simulink model "Copy_of_linkleg_trajectory_contact"  (R2022b)
settings: Solver=daessc  StartTime=0.0  StopTime=4  FixedStep=0.001  MaxStep=0.0025  RelTol=3e-3  AbsTol=3e-3  EnableMultiTasking=on
StopFcn:
  | Initialize = 0;
model workspace (MAT data in the model file):
  Initialize = Simulink.Signal
  Initialize.DataType = 'auto'
  Initialize.Dimensions = -1
  Initialize.DimensionsMode = 'auto'
  Initialize.Complexity = 'auto'
  Initialize.SampleTime = -1
  Initialize.SamplingMode = 'auto'
  Initialize.InitialValue = '0'
  Var = [0; 0; 0]
undefined symbols (not defined in the file or in its folder): X, Y, Z
libraries: sm_lib x86, nesl_utility x18, fl_lib x8, simulink x7, slpidlib x2, Contact_Forces_Lib x1
(part 1 of 3)
settings Model: SimulationMode=accelerator  Creator=guanlunlu  LastModifiedBy=guanlunlu
settings SolverCC: AutoScaleAbsTol=off  InitialStep=0.0025  MaxZcPerStep=1
settings DataIOCC: LimitDataPoints=on  MaxDataPoints=10000  LoggingToFile=on
settings OptimizationCC: DefaultParameterBehavior=Inlined  UseDivisionForNetSlopeComputation=on  GainParamInheritBuiltInType=on  UseFloatMulNetSlope=on  InlineInvariantSignals=on  EfficientFloat2IntCast=on  LifeSpan=1
settings DebuggingCC: UnconnectedInputMsg=warning  UnconnectedOutputMsg=warning  UnconnectedLineMsg=warning  AllowSymbolicDim=off  SFUnexpectedBacktrackingDiag=warning  SFNoUnconditionalDefaultTransitionDiag=warning  SFExecutionAtInitializationDiag=none  SFMachineParentedDataDiag=warning  ArithmeticOperatorsInVariantConditions=warning
settings HardwareCC: ProdLongLongMode=on
settings ModelReferenceCC: EnableRefExpFcnMdlSchedulingChecks=on
settings SFSimCC: SimUseLocalCustomCode=off  MATLABDynamicMemAlloc=off  CustomCodeUndefinedFunction=UseInterfaceOnly
settings RTWCC: GenerateReport=on  RTWUseLocalCustomCode=off  LaunchReport=on  DLArmComputeVersion=19.05
settings CodeAppCC: ForceParamTrailComments=on
settings GRTTargetCC: TargetLangStandard=C89/C90 (ANSI)  CombineSignalStateStructs=on  MatFileLogging=off  SupportVariableSizeSignals=on
settings ConfigComp: CovMetricSettings=dw  CovSaveCumulativeToWorkspaceVar=on  CovSaveSingleToWorkspaceVar=on  CovExternalEMLEnable=off  CovSFcnEnable=off
settings SimscapeCC: SimscapeLogType=all  SimscapeLogSimulationStatistics=on  SimscapeLogDataHistory=10000
settings ExplorerConfigSet: InternalSimMechanicsExplorerSettings="<ExplorerConfiguration><canonicalview>default</canonicalview><AnimationSetting><BasePlaybackSpeed>1.0</BasePlaybackSpeed><PlaybackSpeedFactor>1.0</PlaybackSpeedFactor></AnimationSetting><TilePanel><TileInfo><Tiles Columns=\"1\" Count=\"1\" Rows=\"1\"><Column Weight=\"1\"/><Row Weight=\"1\"/><Tile Height=\"1\" Width=\"1\" X=\"0\" Y=\"0\"/></Tiles></TileInfo><SceneInfo><SceneViewer><BGColor><R>1</R><G>1</G><B>1</B></BGColor><Camera><DoPerspective>off</DoPerspective><Position><X>0.000681433050903873516</X><Y>-0.0104115297967437362</Y><Z>1428355.60663242452</Z></Position><Center><X>0.000681433050903873516</X><Y>-0.0104115297967437362</Y><Z>2.07935910268020052e-07</Z></Center><Up><X>0</X><Y>1</Y><Z>-0</Z></Up><ViewLimDist>1</ViewLimDist><YLim>0.224878371170773472</YLim><XLim>0.312101415871202159</XLim></Camera></SceneViewer></SceneInfo></TilePanel><MechEditorPanel><Cameras/><GfxPanelCameraMap/><VideoCreator><PlaybackSpeedRatio>1.0</PlaybackSpeedRatio><FrameRate>30</FrameRate><VideoFormat>Motion JPEG AVI</VideoFormat><FrameSize>auto</FrameSize></VideoCreator></MechEditorPanel></ExplorerConfiguration>"

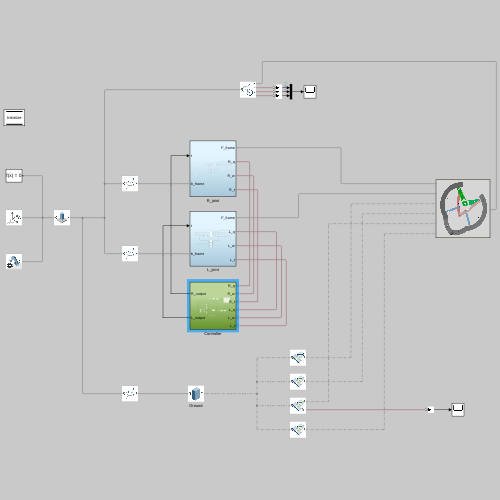
[thumbnail: Simulink's stored preview of the top-level diagram]
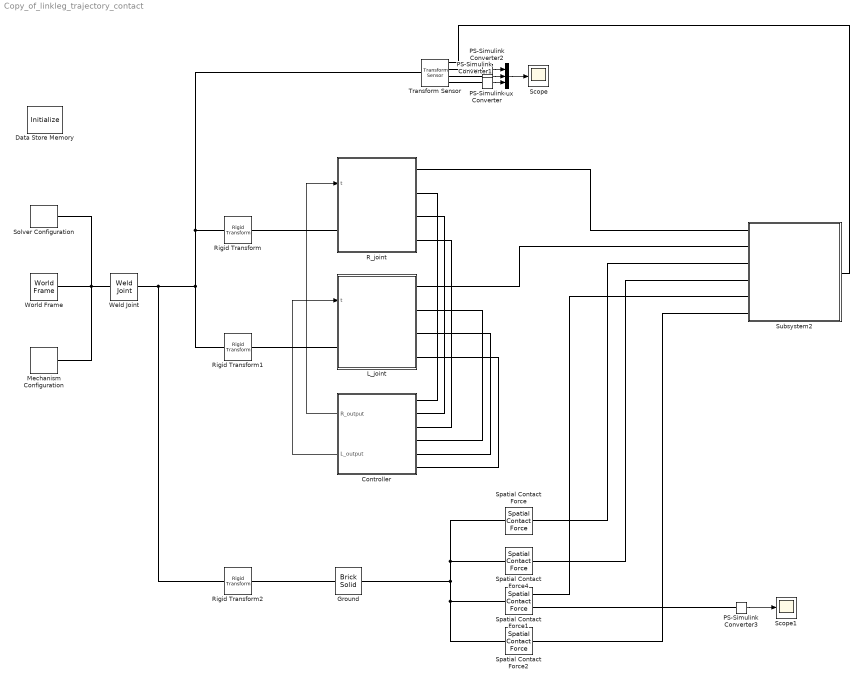
== system Copy_of_linkleg_trajectory_contact ==
  Controller : Subsystem
  Data Store Memory : DataStoreMemory  DataStoreName=Initialize  WriteAfterWriteMsg=warning  ShowAdditionalParam=off  StateMustResolveToSignalObject=on
  Ground : sm_lib/Body Elements/Brick Solid  GraphicAmbientColor=[0.15 0.15 0.15 1.0]  BasedOnType=Density  BrickDimensions=[1 1 0.02]  BrickDimensionUnits=m  CenterOfMass=[0 0 0]  CenterOfMassUnits=m  GraphicDiffuseColor=[1.0 0.8 0.8]  Density=1000  DensityUnits=kg/m^3  DoExposeReferenceFrame=on  GraphicEmissiveColor=[0.0 0.0 0.0 1.0]  ExportEntireGeometry=on  SerializedFrames=<Frames/>  MarkerShape=Sphere  MarkerSize=10  GraphicType=FromGeometry  InertiaType=CalculateFromGeometry  Mass=1  MassUnits=kg  MomentsOfInertia=[1 1 1]  MomentsOfInertiaUnits=kg*m^2  GraphicOpacity=1.0  ProductsOfInertia=[0 0 0]  ProductsOfInertiaUnits=kg*m^2  GraphicShininess=75  GraphicSpecularColor=[0.5 0.5 0.5 1.0]  GraphicVisPropType=SimpleVisualProperties
  L_joint : Subsystem
  Mechanism Configuration : sm_lib/Utilities/Mechanism Configuration  UniformGravity=Constant  GravityVector=[0 -9.80665 0]  GravityUnits=m/s^2  LinearizationDelta=0.001  JointModeTransitionNonlinearIterations=2
  Mux : Mux  Inputs=3
  PS-Simulink Converter{,1..3} (4 alike) : nesl_utility/PS-Simulink Converter  PhysicalDomain=network_engine_domain  SubClassName=ps_output  LeftPortType=input  RightPortType=output  PseudoPeriodic=off  Frequencies=[]  VectorFormat=inherit  Unit=inherit  AffineConversion=off
  R_joint : Subsystem
  Rigid Transform : sm_lib/Frames and Transforms/Rigid Transform  TranslationMethod=Cartesian  TranslationStandardOffset=0  TranslationLengthUnit=m  TranslationStandardAxis=+Z  TranslationCartesianOffset=[0 0 -0.005]  TranslationROffset=0  TranslationROffsetUnits=m  TranslationZOffset=0  TranslationZOffsetUnits=m  TranslationThetaOffset=0  TranslationThetaOffsetUnits=deg  RotationMethod=RotationSequence  RotationAngleUnits=deg  RotationStandardAxis=-Z  RotationAngle=0.0  RotationArbitraryAxis=[0 0 1]  FollAlignAxisA=+X  BaseAlignAxisA=+Y  FollAlignAxisB=+Y  BaseAlignAxisB=+Z  RotationSequenceAxes=FollowerAxes  RotationSequence=XYX  RotationSequenceAngles=[0 0 0]  RotationSequenceAnglesUnits=deg  RotationMatrix=[1 0 0; 0 1 0; 0 0 -1]  Quaternion=[1 0 0 0]
  Rigid Transform1 : sm_lib/Frames and Transforms/Rigid Transform  TranslationMethod=Cartesian  TranslationStandardOffset=0  TranslationLengthUnit=m  TranslationStandardAxis=+Z  TranslationCartesianOffset=[0 0 0.005]  TranslationROffset=0  TranslationROffsetUnits=m  TranslationZOffset=0  TranslationZOffsetUnits=m  TranslationThetaOffset=0  TranslationThetaOffsetUnits=deg  RotationMethod=None  RotationAngleUnits=deg  RotationStandardAxis=+Z  RotationAngle=0.0  RotationArbitraryAxis=[0 0 1]  FollAlignAxisA=+X  BaseAlignAxisA=+Y  FollAlignAxisB=+Y  BaseAlignAxisB=+Z  RotationSequenceAxes=FollowerAxes  RotationSequence=XYX  RotationSequenceAngles=[0 0 0]  RotationSequenceAnglesUnits=deg  RotationMatrix=[1 0 0; 0 1 0; 0 0 1]  Quaternion=[1 0 0 0]
  Rigid Transform2 : sm_lib/Frames and Transforms/Rigid Transform  TranslationMethod=Cartesian  TranslationStandardOffset=0  TranslationLengthUnit=m  TranslationStandardAxis=+Z  TranslationCartesianOffset=[0 -0.21 0]  TranslationROffset=0  TranslationROffsetUnits=m  TranslationZOffset=0  TranslationZOffsetUnits=m  TranslationThetaOffset=0  TranslationThetaOffsetUnits=deg  RotationMethod=StandardAxis  RotationAngleUnits=deg  RotationStandardAxis=-X  RotationAngle=90  RotationArbitraryAxis=[0 0 1]  FollAlignAxisA=+X  BaseAlignAxisA=+Y  FollAlignAxisB=+Y  BaseAlignAxisB=+Z  RotationSequenceAxes=FollowerAxes  RotationSequence=XYX  RotationSequenceAngles=[0 0 0]  RotationSequenceAnglesUnits=deg  RotationMatrix=[1 0 0; 0 1 0; 0 0 1]  Quaternion=[1 0 0 0]
  Scope : Scope
  Scope1 : Scope
  Solver Configuration : nesl_utility/Solver Configuration  PhysicalDomain=network_engine_domain  SubClassName=solver  LeftPortType=input  RightPortType=generic  Tones=[]  Harmonics=[]  SimulateNoise=off  Profile=off  UseLocalSampling=off  EnableSwitchedLinearOptims=on  FrequencyDomain=off  UseCCode=off  RelTol=0.001  AbsTol=1e-06  MinStep=1e-09  ToWorkspace=off  RevertToSquareIcSolve=off  NumHomotopyIterations=100  PhasorMode=off  PhasorModeNumHarmonics=1  ConsistencySolver=NEWTON_XTOL_AFTER_FTOL  IndexReductionMethod=DerivativeReplacement  DoDC=off  ResidualTolerance=1e-09  ConsistencyTolSource=GLOBAL  ConsistencyAbsTol=0.001  ConsistencyRelTol=0.001  ConsistencyTolFactor=0.001  UseLocalSolver=off  LocalSolverChoice=NE_BACKWARD_EULER_ADVANCER  ResolveIndetEquations=on  FunctionEvalNumThread=1  LocalSolverSampleTime=0.001  DoFixedCost=off  MaxNonlinIter=3  MaxModeIter=2  ComputeImpulses=off  ImpulseIterations=2  LinearAlgebra=Sparse  LinearAlgebraNumThread=0  EquationFormulation=NE_TIME_EF  DelaysMemoryBudget=1024  AutomaticFiltering=on  FilteringTimeConstant=0.001  PartitionStorageMethod=AS_NEEDED  PartitionMemoryBudget=1024  PartitionMethod=FAST
  Spatial Contact Force : sm_lib/Forces and Torques/Spatial Contact Force  SenseContactBaseRotation=off  SenseContactBaseTranslation=off  CoefficientOfDynamicFriction=0.2  CoefficientOfStaticFriction=0.2  NormalDamping=contact_dmp  NormalDampingUnits=N/(m/s)  SenseContactSignal=off  NormalStiffness=contact_stf  NormalStiffnessUnits=N/m  FrictionalCriticalVelocity=1e-3  FrictionalCriticalVelocityUnits=m/s  ZeroCrossDetectContactStartAndEnd=off  SenseContactFollowerRotation=off  SenseContactFollowerTranslation=off  FrictionType=SmoothStickSlip  SenseFrictionalForceMagnitude=off  SenseNormalForceMagnitude=off  NormalForceType=SmoothSpringDamper  SenseNormalVelocity=off  SenseSeparationDistance=off  SenseTangentialVelocity=off  NormalTransitionRegionWidth=contact_trs  NormalTransitionRegionWidthUnits=m
  Spatial Contact Force1 : sm_lib/Forces and Torques/Spatial Contact Force  SenseContactBaseRotation=off  SenseContactBaseTranslation=off  CoefficientOfDynamicFriction=0.2  CoefficientOfStaticFriction=0.2  NormalDamping=contact_dmp  NormalDampingUnits=N/(m/s)  SenseContactSignal=off  NormalStiffness=contact_stf  NormalStiffnessUnits=N/m  FrictionalCriticalVelocity=1e-3  FrictionalCriticalVelocityUnits=m/s  ZeroCrossDetectContactStartAndEnd=off  SenseContactFollowerRotation=off  SenseContactFollowerTranslation=off  FrictionType=SmoothStickSlip  SenseFrictionalForceMagnitude=off  SenseNormalForceMagnitude=on  NormalForceType=SmoothSpringDamper  SenseNormalVelocity=off  SenseSeparationDistance=off  SenseTangentialVelocity=off  NormalTransitionRegionWidth=contact_trs  NormalTransitionRegionWidthUnits=m
  Spatial Contact Force2 : sm_lib/Forces and Torques/Spatial Contact Force  SenseContactBaseRotation=off  SenseContactBaseTranslation=off  CoefficientOfDynamicFriction=0.2  CoefficientOfStaticFriction=0.2  NormalDamping=contact_dmp  NormalDampingUnits=N/(m/s)  SenseContactSignal=off  NormalStiffness=contact_stf  NormalStiffnessUnits=N/m  FrictionalCriticalVelocity=1e-3  FrictionalCriticalVelocityUnits=m/s  ZeroCrossDetectContactStartAndEnd=off  SenseContactFollowerRotation=off  SenseContactFollowerTranslation=off  FrictionType=SmoothStickSlip  SenseFrictionalForceMagnitude=off  SenseNormalForceMagnitude=off  NormalForceType=SmoothSpringDamper  SenseNormalVelocity=off  SenseSeparationDistance=off  SenseTangentialVelocity=off  NormalTransitionRegionWidth=contact_trs  NormalTransitionRegionWidthUnits=m
  Spatial Contact Force4 : sm_lib/Forces and Torques/Spatial Contact Force  SenseContactBaseRotation=off  SenseContactBaseTranslation=off  CoefficientOfDynamicFriction=0.2  CoefficientOfStaticFriction=0.2  NormalDamping=contact_dmp  NormalDampingUnits=N/(m/s)  SenseContactSignal=off  NormalStiffness=contact_stf  NormalStiffnessUnits=N/m  FrictionalCriticalVelocity=1e-3  FrictionalCriticalVelocityUnits=m/s  ZeroCrossDetectContactStartAndEnd=off  SenseContactFollowerRotation=off  SenseContactFollowerTranslation=off  FrictionType=SmoothStickSlip  SenseFrictionalForceMagnitude=off  SenseNormalForceMagnitude=off  NormalForceType=SmoothSpringDamper  SenseNormalVelocity=off  SenseSeparationDistance=off  SenseTangentialVelocity=off  NormalTransitionRegionWidth=contact_trs  NormalTransitionRegionWidthUnits=m
  Subsystem2 : Subsystem
      mask Display: image('$imagefile'); % Use "Edit Image" on toolstrip to change.
  Transform Sensor : sm_lib/Frames and Transforms/Transform Sensor  MeasurementFrame=World  SenseAngle=off  SenseAxis=off  SenseQ=off  SenseR=off  SenseRotationSequence=off  RotationSequence=XYX  SenseOmegaX=off  SenseOmegaY=off  SenseOmegaZ=off  SenseQDot=off  SenseRDot=off  SenseAlphaX=off  SenseAlphaY=off  SenseAlphaZ=off  SenseQDDot=off  SenseRDDot=off  SenseX=on  SenseY=on  SenseZ=on  SenseRad=off  SenseAzim=off  SenseDist=off  SenseInc=off  SenseXDot=off  SenseYDot=off  SenseZDot=off  SenseRadDot=off  SenseAzimDot=off  SenseDistDot=off  SenseIncDot=off  SenseXDDot=off  SenseYDDot=off  SenseZDDot=off  SenseRadDDot=off  SenseAzimDDot=off  SenseDistDDot=off  SenseIncDDot=off
  Weld Joint : sm_lib/Joints/Weld Joint  JointMode=Normal  SenseConstraintForce=off  SenseConstraintForceX=off  SenseConstraintForceY=off  SenseConstraintForceZ=off  SenseConstraintTorque=off  SenseConstraintTorqueX=off  SenseConstraintTorqueY=off  SenseConstraintTorqueZ=off  SenseTotalForce=off  SenseTotalForceX=off  SenseTotalForceY=off  SenseTotalForceZ=off  SenseTotalTorque=off  SenseTotalTorqueX=off  SenseTotalTorqueY=off  SenseTotalTorqueZ=off  CompositeWrenchDir=FollowerOnBase  CompositeWrenchFrame=BaseFrame
  World Frame : sm_lib/Frames and Transforms/World Frame
  wires:
  Controller/1(R_output) -> R_joint/1(t)
  Controller/2(L_output) -> L_joint/1(t)
  Mux/1 -> Scope/1
  PS-Simulink Converter2/1 -> Mux/1
  PS-Simulink Converter1/1 -> Mux/3
  PS-Simulink Converter/1 -> Mux/2
  PS-Simulink Converter3/1 -> Scope1/1
  connections:
  World Frame/RConn1 -- Mechanism Configuration/RConn1 -- Weld Joint/LConn1 -- Solver Configuration/RConn1
  Rigid Transform/LConn1 -- Transform Sensor/LConn1 -- Rigid Transform1/LConn1 -- Rigid Transform2/LConn1 -- Weld Joint/RConn1
  Ground/RConn1 -- Rigid Transform2/RConn1
  R_joint/LConn1 -- Rigid Transform/RConn1
  Rigid Transform1/RConn1 -- L_joint/LConn1
  R_joint/RConn1 -- Subsystem2/LConn1
  L_joint/RConn1 -- Subsystem2/LConn2
  Spatial Contact Force/LConn1 -- Spatial Contact Force4/LConn1 -- Spatial Contact Force2/LConn1 -- Spatial Contact Force1/LConn1 -- Ground/LConn1
  Spatial Contact Force4/RConn1 -- Subsystem2/LConn4
  Spatial Contact Force/RConn1 -- Subsystem2/LConn3
  Spatial Contact Force1/RConn1 -- Subsystem2/LConn5
  Spatial Contact Force2/RConn1 -- Subsystem2/LConn6
  R_joint/RConn2 -- Controller/LConn1
  R_joint/RConn3 -- Controller/LConn2
  R_joint/RConn4 -- Controller/LConn3
  L_joint/RConn2 -- Controller/LConn4
  L_joint/RConn3 -- Controller/LConn5
  L_joint/RConn4 -- Controller/LConn6
  Transform Sensor/RConn1 -- Subsystem2/RConn1
  PS-Simulink Converter2/LConn1 -- Transform Sensor/RConn2
  Transform Sensor/RConn3 -- PS-Simulink Converter/LConn1
  Transform Sensor/RConn4 -- PS-Simulink Converter1/LConn1
  PS-Simulink Converter3/LConn1 -- Spatial Contact Force1/RConn2

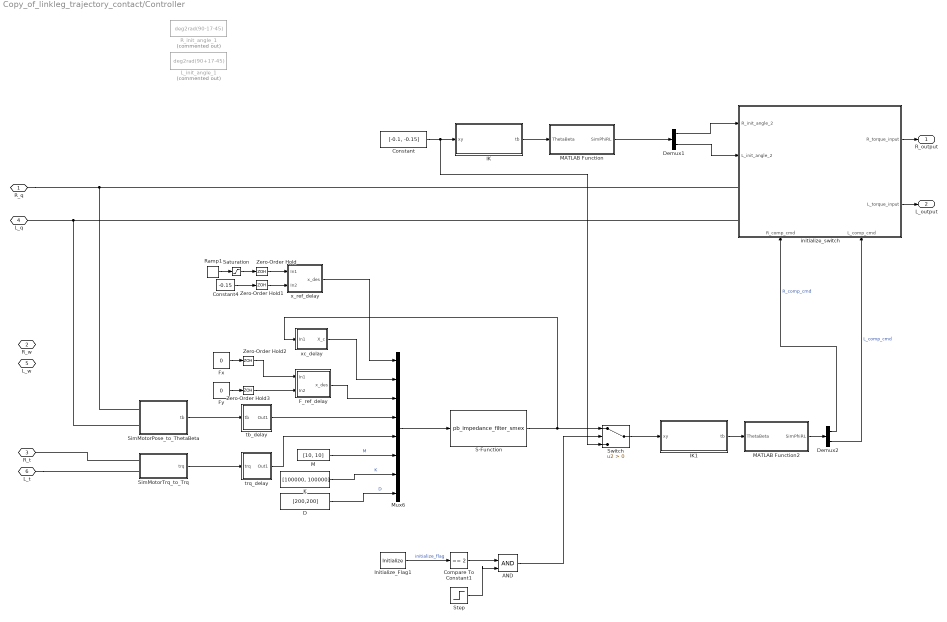
== system Copy_of_linkleg_trajectory_contact/Controller ==
  AND : Logic  IconShape=distinctive  AllPortsSameDT=off  OutDataTypeStr=boolean
  Compare To Constant1 : simulink/Logic and Bit Operations/Compare To Constant  relop===  const=2  OutDataTypeStr=uint8
  Constant : Constant  Value=[-0.1, -0.15]
  Constant4 : Constant  Value=-0.15
  D : Constant  Value=[200,200]
  Demux1 : Demux  Outputs=2
  Demux2 : Demux  Outputs=2
  F_ref_delay : Subsystem
  Fx : Constant  Value=0
  Fy : Constant  Value=0
  IK : MATLAB Function  TreatAsAtomicUnit=on
  IK1 : MATLAB Function  TreatAsAtomicUnit=on
  Initialize_Flag1 : DataStoreRead  DataStoreName=Initialize  IndexOptions=Index vector (dialog)  Indices=1  OutputSizes=1
  K : Constant  Value=[100000, 100000]
  L_init_angle_1 : Constant  Commented=on  Value=deg2rad(90+17-45)
  M : Constant  Value=[10, 10]
  MATLAB Function : MATLAB Function  TreatAsAtomicUnit=on
  MATLAB Function2 : MATLAB Function  TreatAsAtomicUnit=on
  Mux6 : Mux  Inputs=8
  R_init_angle_1 : Constant  Commented=on  Value=deg2rad(90-17-45)
  Ramp1 : simulink/Sources/Ramp  slope=0.1  start=1  InitialOutput=-0.1
  S-Function : S-Function  FunctionName=pb_impedance_filter_smex  SFunctionDeploymentMode=off  EnableBusSupport=off
  Saturation : Saturate  UpperLimit=0.1
  SimMotorPose_to_ThetaBeta : Subsystem
  SimMotorTrq_to_Trq : Subsystem
  Step : Step  SampleTime=0
  Switch : Switch  Criteria=u2 > Threshold  SaturateOnIntegerOverflow=off  InputSameDT=off
  Zero-Order Hold{,1..3} (4 alike) : ZeroOrderHold  SampleTime=-1
  initialize_switch : Subsystem
      settings: PortSchema="{\"entries\":[{\"content\":{\"sides\":[{\"content\":{\"connectorIds\":[\"In1\",\"In2\",\"LConn1\",\"LConn2\"]},\"type\":\"ConnectorPlacement.EquallySpacedRectSide\",\"uuid\":\"90e40c7c-5865-4836-be41-da90a1037084\"},{\"content\":{\"connectorIds\":[\"Out1\",\"Out2\"],\"side\":\"RIGHT\"},\"type\":\"ConnectorPlacement.EquallySpacedRectSide\",\"uuid\":\"b839b53b-6c19-45bc-b89b-7b093b626138\"},{\"content\":{\"connectorIds\":[],\"side\":\"TOP\"},\"type\":\"ConnectorPlacement.EquallySpacedRectSide\",\"uuid\":\"45e31397-8701-4b08-8e72-be675cbdf183\"},{\"content\":{\"connectorIds\":[\"In3\",\"In4\"],\"side\":\"BOTTOM\"},\"type\":\"ConnectorPlacement.EquallySpacedRectSide\",\"uuid\":\"48276d5b-6512-4d04-ace7-a3d739604563\"}]},\"type\":\"ConnectorPlacement.EquallySpacedConnector\",\"uuid\":\"ed524fdc-357c-4d9e-8bf8-882e26daba64\"}],\"packageUris\":[\"http://schema.mathworks.com/mf0/Connector/R2020b\"],\"version\":\"1.0\"}"
  tb_delay : Subsystem
  trq_delay : Subsystem
  x_ref_delay : Subsystem
  xc_delay : Subsystem
  R_q : PMIOPort  Side=Left
  R_w : PMIOPort  Port=2  Side=Left
  R_t : PMIOPort  Port=3  Side=Left
  L_q : PMIOPort  Port=4  Side=Left
  L_w : PMIOPort  Port=5  Side=Left
  L_t : PMIOPort  Port=6  Side=Left
  R_output : Outport
  L_output : Outport  Port=2
  wires:
  initialize_switch/2(L_torque_input) -> L_output/1
  Demux1/2 -> initialize_switch/2(L_init_angle_2)
  initialize_switch/1(R_torque_input) -> R_output/1
  Demux1/1 -> initialize_switch/1(R_init_angle_2)
  Constant/1 -> Switch/3, IK/1(xy)
  IK/1(tb) -> MATLAB Function/1(ThetaBeta)
  MATLAB Function/1(SimPhiRL) -> Demux1/1
  Fy/1 -> Zero-Order Hold3/1
  Ramp1/1 -> Saturation/1
  tb_delay/1(Out1) -> Mux6/4
  MATLAB Function2/1(SimPhiRL) -> Demux2/1
  Mux6/1 -> S-Function/1
  IK1/1(tb) -> MATLAB Function2/1(ThetaBeta)
  Fx/1 -> Zero-Order Hold2/1
  F_ref_delay/1(x_des) -> Mux6/3
  trq_delay/1(Out1) -> Mux6/5
  x_ref_delay/1(x_des) -> Mux6/1
  K/1 -> Mux6/7  "K"
  M/1 -> Mux6/6  "M"
  Constant4/1 -> Zero-Order Hold1/1
  D/1 -> Mux6/8  "D"
  xc_delay/1(X_c) -> Mux6/2
  Demux2/1 -> initialize_switch/3(R_comp_cmd)  "R_comp_cmd"
  Demux2/2 -> initialize_switch/4(L_comp_cmd)  "L_comp_cmd"
  SimMotorPose_to_ThetaBeta/1(tb) -> tb_delay/1(tb)
  SimMotorTrq_to_Trq/1(trq) -> trq_delay/1(trq)
  S-Function/1 -> xc_delay/1(In1), Switch/1
  AND/1 -> Switch/2
  Switch/1 -> IK1/1(xy)
  Step/1 -> AND/2
  Initialize_Flag1/1 -> Compare To Constant1/1  "initialize_flag"
  Compare To Constant1/1 -> AND/1
  Zero-Order Hold/1 -> x_ref_delay/1(In1)
  Zero-Order Hold1/1 -> x_ref_delay/2(In2)
  Zero-Order Hold2/1 -> F_ref_delay/1(In1)
  Zero-Order Hold3/1 -> F_ref_delay/2(In2)
  Saturation/1 -> Zero-Order Hold/1
  connections:
  R_q/RConn1 -- SimMotorPose_to_ThetaBeta/LConn1 -- initialize_switch/LConn1
  initialize_switch/LConn2 -- SimMotorPose_to_ThetaBeta/LConn2 -- L_q/RConn1
  L_t/RConn1 -- SimMotorTrq_to_Trq/LConn2
  SimMotorTrq_to_Trq/LConn1 -- R_t/RConn1

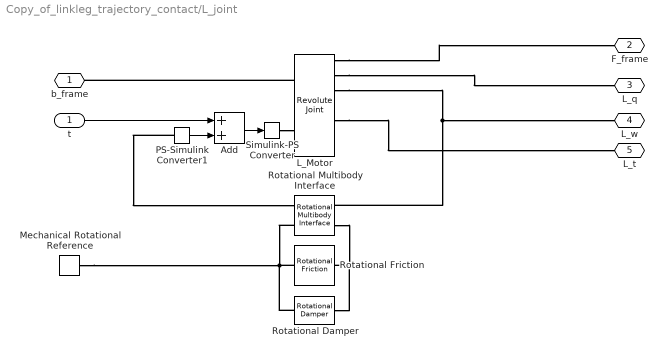
== system Copy_of_linkleg_trajectory_contact/L_joint ==
  t : Inport
  Add : Sum
  L_Motor : sm_lib/Joints/Revolute Joint  JointMode=Normal  SenseConstraintForce=on  SenseConstraintForceX=off  SenseConstraintForceY=off  SenseConstraintForceZ=off  SenseConstraintTorque=on  SenseConstraintTorqueX=off  SenseConstraintTorqueY=off  SenseConstraintTorqueZ=off  SenseTotalForce=off  SenseTotalForceX=off  SenseTotalForceY=off  SenseTotalForceZ=off  SenseTotalTorque=off  SenseTotalTorqueX=off  SenseTotalTorqueY=off  SenseTotalTorqueZ=off  CompositeWrenchDir=FollowerOnBase  CompositeWrenchFrame=BaseFrame  EquilibriumPosition=0  EquilibriumPositionUnits=deg  SpringStiffness=0  SpringStiffnessUnits=N*m/deg  DampingCoefficient=0  DampingCoefficientUnits=N*m/(rad/s)  TorqueActuationMode=InputTorque  MotionActuationMode=ComputedMotion  SensePosition=on  SenseVelocity=on  SenseAcceleration=on  SenseTorqueForce=on  SenseLowerLimitTorqueForce=off  SenseUpperLimitTorqueForce=off  LowerLimitSpecify=off  LowerLimitBound=-90  LowerLimitBoundUnits=deg  LowerLimitStiffness=1e4  LowerLimitStiffnessUnits=N*m/deg  LowerLimitDamping=10  LowerLimitDampingUnits=N*m/(deg/s)  LowerLimitTransitionRegionWidth=0.1  LowerLimitTransitionRegionWidthUnits=deg  UpperLimitSpecify=off  UpperLimitBound=90  UpperLimitBoundUnits=deg  UpperLimitStiffness=1e4  UpperLimitStiffnessUnits=N*m/deg  UpperLimitDamping=10  UpperLimitDampingUnits=N*m/(deg/s)  UpperLimitTransitionRegionWidth=0.1  UpperLimitTransitionRegionWidthUnits=deg  PositionTargetSpecify=on  PositionTargetPriority=High  PositionTargetValue=160  PositionTargetValueUnits=deg  VelocityTargetSpecify=off  VelocityTargetPriority=High  VelocityTargetValue=0  VelocityTargetValueUnits=deg/s
  Mechanical Rotational Reference : fl_lib/Mechanical/Rotational Elements/Mechanical Rotational Reference
  PS-Simulink Converter1 : nesl_utility/PS-Simulink Converter  PhysicalDomain=network_engine_domain  SubClassName=ps_output  LeftPortType=input  RightPortType=output  PseudoPeriodic=off  Frequencies=[]  VectorFormat=inherit  Unit=inherit  AffineConversion=off
  Rotational Damper : fl_lib/Mechanical/Rotational Elements/Rotational Damper  D=0.05 N*m*s/rad  w_specify=off  w_priority=None  w=0 rad/s  w_nominal_specify=off  w_nominal_unit=rad/s  w_nominal_value=1  t_specify=off  t_priority=None  t=0 N*m  t_nominal_specify=off  t_nominal_unit=N*m  t_nominal_value=1
  Rotational Friction : fl_lib/Mechanical/Rotational Elements/Rotational Friction  brkwy_trq=bk_ft N*m  brkwy_vel=bk_vel rad/s  Col_trq=col_ft N*m  visc_coef=vis_ft N*m*s/rad  w_specify=on  w_priority=None  w=0 rad/s  w_nominal_specify=off  w_nominal_unit=rad/s  w_nominal_value=1  t_specify=on  t_priority=None  t=0 N*m  t_nominal_specify=off  t_nominal_unit=N*m  t_nominal_value=1
  Rotational Multibody Interface : fl_lib/Mechanical/Multibody Interfaces/Rotational Multibody Interface
  Simulink-PS Converter : nesl_utility/Simulink-PS Converter  PhysicalDomain=network_engine_domain  SubClassName=ps_input  LeftPortType=input  RightPortType=output  PseudoPeriodic=off  Frequencies=[]  NoiseDistribution=none  NoiseParameters=[]  Unit=1  AffineConversion=off  FilteringAndDerivatives=provide  SimscapeFilterOrder=1  InputFilterTimeConstant=0.001  UdotUserProvided=0
  b_frame : PMIOPort  Side=Left
  F_frame : PMIOPort  Port=2  Side=Right
  L_q : PMIOPort  Port=3  Side=Right
  L_w : PMIOPort  Port=4  Side=Right
  L_t : PMIOPort  Port=5  Side=Right
  wires:
  PS-Simulink Converter1/1 -> Add/2
  Add/1 -> Simulink-PS Converter/1
  t/1 -> Add/1
  connections:
  PS-Simulink Converter1/LConn1 -- Rotational Multibody Interface/LConn1
  L_Motor/RConn1 -- F_frame/RConn1
  L_Motor/LConn1 -- b_frame/RConn1
  Rotational Multibody Interface/RConn2 -- Rotational Damper/LConn1 -- Rotational Friction/LConn1
  Simulink-PS Converter/RConn1 -- L_Motor/LConn2
  Rotational Multibody Interface/LConn2 -- Mechanical Rotational Reference/LConn1 -- Rotational Damper/RConn1 -- Rotational Friction/RConn1
  L_Motor/RConn3 -- L_w/RConn1 -- Rotational Multibody Interface/RConn1
  L_Motor/RConn2 -- L_q/RConn1
  L_Motor/RConn5 -- L_t/RConn1

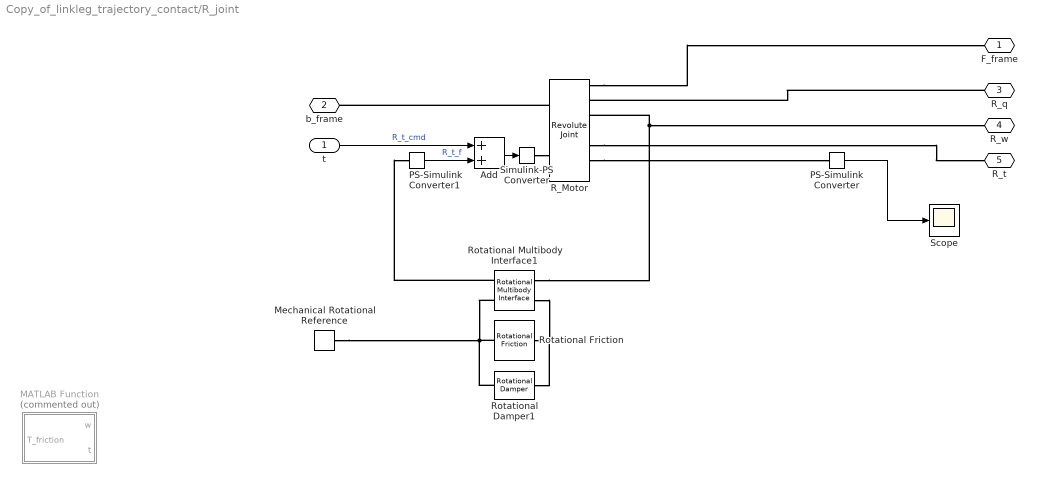
== system Copy_of_linkleg_trajectory_contact/R_joint ==
  t : Inport
  Add : Sum
  MATLAB Function : MATLAB Function  Commented=on  TreatAsAtomicUnit=on
  Mechanical Rotational Reference : fl_lib/Mechanical/Rotational Elements/Mechanical Rotational Reference
  PS-Simulink Converter : nesl_utility/PS-Simulink Converter  PhysicalDomain=network_engine_domain  SubClassName=ps_output  LeftPortType=input  RightPortType=output  PseudoPeriodic=off  Frequencies=[]  VectorFormat=inherit  Unit=inherit  AffineConversion=off
  PS-Simulink Converter1 : nesl_utility/PS-Simulink Converter  PhysicalDomain=network_engine_domain  SubClassName=ps_output  LeftPortType=input  RightPortType=output  PseudoPeriodic=off  Frequencies=[]  VectorFormat=inherit  Unit=inherit  AffineConversion=off
  R_Motor : sm_lib/Joints/Revolute Joint  JointMode=Normal  SenseConstraintForce=on  SenseConstraintForceX=off  SenseConstraintForceY=off  SenseConstraintForceZ=off  SenseConstraintTorque=on  SenseConstraintTorqueX=off  SenseConstraintTorqueY=off  SenseConstraintTorqueZ=off  SenseTotalForce=off  SenseTotalForceX=off  SenseTotalForceY=off  SenseTotalForceZ=off  SenseTotalTorque=off  SenseTotalTorqueX=off  SenseTotalTorqueY=off  SenseTotalTorqueZ=off  CompositeWrenchDir=FollowerOnBase  CompositeWrenchFrame=BaseFrame  EquilibriumPosition=0  EquilibriumPositionUnits=deg  SpringStiffness=0  SpringStiffnessUnits=N*m/deg  DampingCoefficient=0  DampingCoefficientUnits=N*m/(rad/s)  TorqueActuationMode=InputTorque  MotionActuationMode=ComputedMotion  SensePosition=on  SenseVelocity=on  SenseAcceleration=on  SenseTorqueForce=on  SenseLowerLimitTorqueForce=off  SenseUpperLimitTorqueForce=off  LowerLimitSpecify=off  LowerLimitBound=-90  LowerLimitBoundUnits=deg  LowerLimitStiffness=1e4  LowerLimitStiffnessUnits=N*m/deg  LowerLimitDamping=10  LowerLimitDampingUnits=N*m/(deg/s)  LowerLimitTransitionRegionWidth=0.1  LowerLimitTransitionRegionWidthUnits=deg  UpperLimitSpecify=off  UpperLimitBound=90  UpperLimitBoundUnits=deg  UpperLimitStiffness=1e4  UpperLimitStiffnessUnits=N*m/deg  UpperLimitDamping=10  UpperLimitDampingUnits=N*m/(deg/s)  UpperLimitTransitionRegionWidth=0.1  UpperLimitTransitionRegionWidthUnits=deg  PositionTargetSpecify=on  PositionTargetPriority=High  PositionTargetValue=-160  PositionTargetValueUnits=deg  VelocityTargetSpecify=off  VelocityTargetPriority=High  VelocityTargetValue=0  VelocityTargetValueUnits=deg/s
  Rotational Damper1 : fl_lib/Mechanical/Rotational Elements/Rotational Damper  D=0.05 N*m*s/rad  w_specify=off  w_priority=None  w=0 rad/s  w_nominal_specify=off  w_nominal_unit=rad/s  w_nominal_value=1  t_specify=off  t_priority=None  t=0 N*m  t_nominal_specify=off  t_nominal_unit=N*m  t_nominal_value=1
  Rotational Friction : fl_lib/Mechanical/Rotational Elements/Rotational Friction  brkwy_trq=bk_ft N*m  brkwy_vel=bk_vel rad/s  Col_trq=col_ft N*m  visc_coef=vis_ft N*m*s/rad  w_specify=on  w_priority=None  w=0 rad/s  w_nominal_specify=off  w_nominal_unit=rad/s  w_nominal_value=1  t_specify=on  t_priority=None  t=0 N*m  t_nominal_specify=off  t_nominal_unit=N*m  t_nominal_value=1
  Rotational Multibody Interface1 : fl_lib/Mechanical/Multibody Interfaces/Rotational Multibody Interface
  Scope : Scope
  Simulink-PS Converter : nesl_utility/Simulink-PS Converter  PhysicalDomain=network_engine_domain  SubClassName=ps_input  LeftPortType=input  RightPortType=output  PseudoPeriodic=off  Frequencies=[]  NoiseDistribution=none  NoiseParameters=[]  Unit=1  AffineConversion=off  FilteringAndDerivatives=provide  SimscapeFilterOrder=1  InputFilterTimeConstant=0.001  UdotUserProvided=0
  F_frame : PMIOPort  Side=Right
  b_frame : PMIOPort  Port=2  Side=Left
  R_q : PMIOPort  Port=3  Side=Right
  R_w : PMIOPort  Port=4  Side=Right
  R_t : PMIOPort  Port=5  Side=Right
  wires:
  Add/1 -> Simulink-PS Converter/1
  PS-Simulink Converter1/1 -> Add/2  "R_t_f"
  t/1 -> Add/1  "R_t_cmd"
  PS-Simulink Converter/1 -> Scope/1
  connections:
  Rotational Multibody Interface1/RConn1 -- R_Motor/RConn3 -- R_w/RConn1
  Simulink-PS Converter/RConn1 -- R_Motor/LConn2
  R_Motor/LConn1 -- b_frame/RConn1
  R_Motor/RConn1 -- F_frame/RConn1
  R_q/RConn1 -- R_Motor/RConn2
  Rotational Multibody Interface1/LConn1 -- PS-Simulink Converter1/LConn1
  Rotational Multibody Interface1/RConn2 -- Rotational Friction/LConn1 -- Rotational Damper1/LConn1
  Mechanical Rotational Reference/LConn1 -- Rotational Friction/RConn1 -- Rotational Damper1/RConn1 -- Rotational Multibody Interface1/LConn2
  R_Motor/RConn6 -- PS-Simulink Converter/LConn1
  R_Motor/RConn5 -- R_t/RConn1

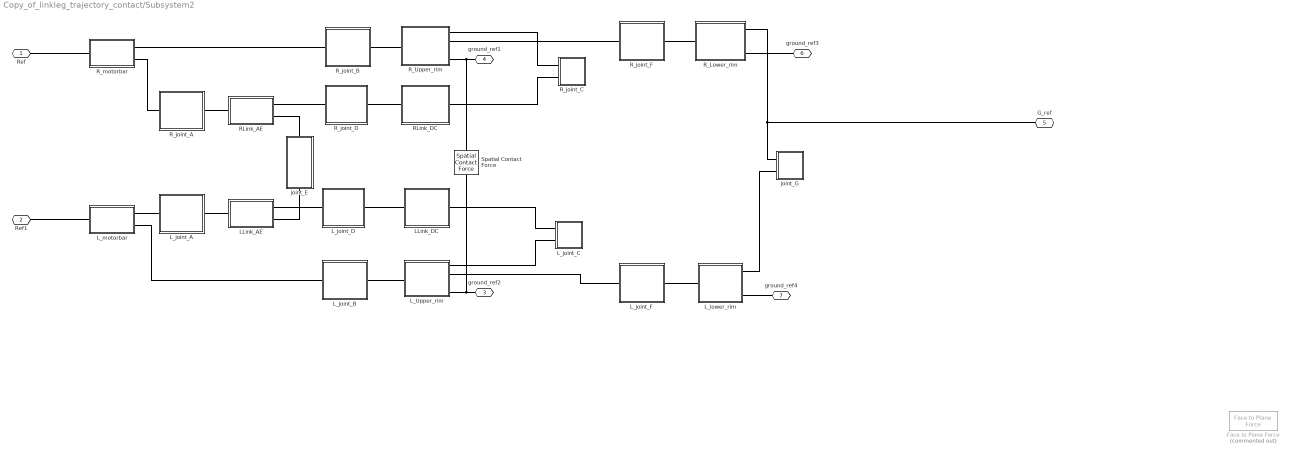
== system Copy_of_linkleg_trajectory_contact/Subsystem2 ==
  Face to Plane Force : Contact_Forces_Lib/3D/Composite Forces/Face to Plane Force  Commented=on  PlaB_x=1  PlaB_y=1  PlaB_z=0.05  FacF_x=0.1  FacF_y=0.1  FacF_z=0.05  FacF_rSph=0.01  force_law_pla2pla=Linear  k_contact_pla2pla=1e4  b_contact_pla2pla=1e2  pen_full_damp_F_pla2pla=1e-4  pen_exponent_pla2pla=1  friction_law_pla2pla=None  mu_kinetic_pla2pla=0.5  mu_static_pla2pla=0.7  v_thr_pla2pla=0.001  vis_on_pla2pla=off  vis_opc_en_box2box=0  vis_len_plaLz=0.005  vis_clr=[0.9 0.2 0.2]  vis_opc=0.7
  LLink_AE : Subsystem
  LLink_DC : Subsystem
  L_Upper_rim : Subsystem
  L_joint_A : Subsystem
  L_joint_B : Subsystem
  L_joint_C : Subsystem
  L_joint_D : Subsystem
  L_joint_F : Subsystem
  L_lower_rim : Subsystem
  L_motorbar : Subsystem
  RLink_AE : Subsystem
  RLink_DC : Subsystem
  R_Lower_rim : Subsystem
  R_Upper_rim : Subsystem
  R_joint_A : Subsystem
  R_joint_B : Subsystem
  R_joint_C : Subsystem
  R_joint_D : Subsystem
  R_joint_F : Subsystem
  R_motorbar : Subsystem
  Spatial Contact Force : sm_lib/Forces and Torques/Spatial Contact Force  SenseContactBaseRotation=off  SenseContactBaseTranslation=off  CoefficientOfDynamicFriction=0.3  CoefficientOfStaticFriction=0.5  NormalDamping=1e3  NormalDampingUnits=N/(m/s)  SenseContactSignal=off  NormalStiffness=1e6  NormalStiffnessUnits=N/m  FrictionalCriticalVelocity=1e-3  FrictionalCriticalVelocityUnits=m/s  ZeroCrossDetectContactStartAndEnd=off  SenseContactFollowerRotation=off  SenseContactFollowerTranslation=off  FrictionType=SmoothStickSlip  SenseFrictionalForceMagnitude=off  SenseNormalForceMagnitude=off  NormalForceType=SmoothSpringDamper  SenseNormalVelocity=off  SenseSeparationDistance=off  SenseTangentialVelocity=off  NormalTransitionRegionWidth=1e-4  NormalTransitionRegionWidthUnits=m
  joint_E : Subsystem
      settings: PortSchema="{\"entries\":[{\"content\":{\"sides\":[{\"content\":{\"connectorIds\":[]},\"type\":\"ConnectorPlacement.EquallySpacedRectSide\",\"uuid\":\"e3540700-35d1-4f33-a6a6-43bad226020a\"},{\"content\":{\"connectorIds\":[],\"side\":\"RIGHT\"},\"type\":\"ConnectorPlacement.EquallySpacedRectSide\",\"uuid\":\"7a9c3a2a-7cba-4d52-8d76-252f342d638f\"},{\"content\":{\"connectorIds\":[\"LConn1\"],\"side\":\"TOP\"},\"type\":\"ConnectorPlacement.EquallySpacedRectSide\",\"uuid\":\"b402f3ac-9bb2-4099-9a28-18a134487b56\"},{\"content\":{\"connectorIds\":[\"RConn1\"],\"side\":\"BOTTOM\"},\"type\":\"ConnectorPlacement.EquallySpacedRectSide\",\"uuid\":\"ad7cac10-3582-47f6-b363-825f8562eb5d\"}]},\"type\":\"ConnectorPlacement.EquallySpacedConnector\",\"uuid\":\"07b66ba2-1ba7-465d-8420-923cb7cf3454\"}],\"packageUris\":[\"http://schema.mathworks.com/mf0/Connector/R2020b\"],\"version\":\"1.0\"}"
  joint_G : Subsystem
  Ref : PMIOPort  Side=Left
  Ref1 : PMIOPort  Port=2  Side=Left
  ground_ref2 : PMIOPort  Port=3  Side=Left
  ground_ref1 : PMIOPort  Port=4  Side=Left
  G_ref : PMIOPort  Port=5  Side=Right
  ground_ref3 : PMIOPort  Port=6  Side=Left
  ground_ref4 : PMIOPort  Port=7  Side=Left
  connections:
  R_motorbar/RConn1 -- R_joint_B/LConn1
  R_Upper_rim/RConn2 -- R_joint_F/LConn1
  LLink_AE/RConn1 -- L_joint_D/LConn1
  R_joint_A/RConn1 -- RLink_AE/LConn1
  joint_G/LConn2 -- L_lower_rim/RConn1
  R_Lower_rim/RConn1 -- G_ref/RConn1 -- joint_G/LConn1
  L_joint_C/LConn1 -- LLink_DC/RConn1
  L_joint_A/LConn1 -- L_motorbar/RConn1
  RLink_AE/RConn2 -- joint_E/LConn1
  R_Upper_rim/LConn1 -- R_joint_B/RConn1
  L_Upper_rim/RConn1 -- L_joint_C/LConn2
  Ref/RConn1 -- R_motorbar/LConn1
  RLink_DC/RConn1 -- R_joint_C/LConn2
  L_joint_A/RConn1 -- LLink_AE/LConn1
  R_motorbar/RConn2 -- R_joint_A/LConn1
  joint_E/RConn1 -- LLink_AE/RConn2
  R_Upper_rim/RConn1 -- R_joint_C/LConn1
  R_joint_D/LConn1 -- RLink_AE/RConn1
  L_joint_D/RConn1 -- LLink_DC/LConn1
  R_joint_F/RConn1 -- R_Lower_rim/LConn1
  RLink_DC/LConn1 -- R_joint_D/RConn1
  L_motorbar/RConn2 -- L_joint_B/LConn1
  L_lower_rim/LConn1 -- L_joint_F/RConn1
  L_joint_F/LConn1 -- L_Upper_rim/RConn2
  L_Upper_rim/LConn1 -- L_joint_B/RConn1
  Ref1/RConn1 -- L_motorbar/LConn1
  ground_ref1/RConn1 -- Spatial Contact Force/LConn1 -- R_Upper_rim/RConn4
  ground_ref2/RConn1 -- L_Upper_rim/RConn4 -- Spatial Contact Force/RConn1
  ground_ref3/RConn1 -- R_Lower_rim/RConn3
  ground_ref4/RConn1 -- L_lower_rim/RConn3

== system Copy_of_linkleg_trajectory_contact/Controller/F_ref_delay ==
  In1 : Inport
  In2 : Inport  Port=2
  Delay : Delay
  Delay1 : Delay
  Delay2 : Delay  DelayLength=1
  Delay3 : Delay  DelayLength=1
  Mux2 : Mux  Inputs=6
  x_des : Outport
  wires:
  In1/1 -> Mux2/1, Delay3/1, Delay/1
  In2/1 -> Mux2/2, Delay2/1, Delay1/1
  Delay2/1 -> Mux2/4
  Delay/1 -> Mux2/5
  Delay3/1 -> Mux2/3
  Mux2/1 -> x_des/1  "x_des"
  Delay1/1 -> Mux2/6

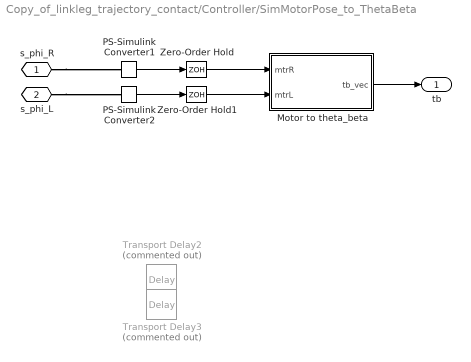
== system Copy_of_linkleg_trajectory_contact/Controller/SimMotorPose_to_ThetaBeta ==
  Motor to theta_beta : MATLAB Function  TreatAsAtomicUnit=on
  PS-Simulink Converter1 : nesl_utility/PS-Simulink Converter  PhysicalDomain=network_engine_domain  SubClassName=ps_output  LeftPortType=input  RightPortType=output  PseudoPeriodic=off  Frequencies=[]  VectorFormat=inherit  Unit=inherit  AffineConversion=off
  PS-Simulink Converter2 : nesl_utility/PS-Simulink Converter  PhysicalDomain=network_engine_domain  SubClassName=ps_output  LeftPortType=input  RightPortType=output  PseudoPeriodic=off  Frequencies=[]  VectorFormat=inherit  Unit=inherit  AffineConversion=off
  Transport Delay2 : TransportDelay  Commented=on  InitialOutput=-0.341
  Transport Delay3 : TransportDelay  Commented=on  InitialOutput=2.51
  Zero-Order Hold : ZeroOrderHold  SampleTime=-1
  Zero-Order Hold1 : ZeroOrderHold  SampleTime=-1
  s_phi_R : PMIOPort  Side=Left
  s_phi_L : PMIOPort  Port=2  Side=Left
  tb : Outport
  wires:
  Motor to theta_beta/1(tb_vec) -> tb/1
  PS-Simulink Converter1/1 -> Zero-Order Hold/1
  PS-Simulink Converter2/1 -> Zero-Order Hold1/1
  Zero-Order Hold1/1 -> Motor to theta_beta/2(mtrL)
  Zero-Order Hold/1 -> Motor to theta_beta/1(mtrR)
  connections:
  s_phi_R/RConn1 -- PS-Simulink Converter1/LConn1
  s_phi_L/RConn1 -- PS-Simulink Converter2/LConn1

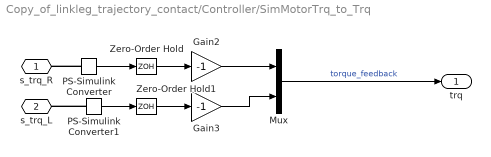
== system Copy_of_linkleg_trajectory_contact/Controller/SimMotorTrq_to_Trq ==
  Gain2 : Gain  Gain=-1
  Gain3 : Gain  Gain=-1
  Mux : Mux  Inputs=2
  PS-Simulink Converter : nesl_utility/PS-Simulink Converter  PhysicalDomain=network_engine_domain  SubClassName=ps_output  LeftPortType=input  RightPortType=output  PseudoPeriodic=off  Frequencies=[]  VectorFormat=inherit  Unit=inherit  AffineConversion=off
  PS-Simulink Converter1 : nesl_utility/PS-Simulink Converter  PhysicalDomain=network_engine_domain  SubClassName=ps_output  LeftPortType=input  RightPortType=output  PseudoPeriodic=off  Frequencies=[]  VectorFormat=inherit  Unit=inherit  AffineConversion=off
  Zero-Order Hold : ZeroOrderHold  SampleTime=-1
  Zero-Order Hold1 : ZeroOrderHold  SampleTime=-1
  s_trq_R : PMIOPort  Side=Left
  s_trq_L : PMIOPort  Port=2  Side=Left
  trq : Outport
  wires:
  Gain2/1 -> Mux/1
  Gain3/1 -> Mux/2
  Mux/1 -> trq/1  "torque_feedback"
  PS-Simulink Converter/1 -> Zero-Order Hold/1
  PS-Simulink Converter1/1 -> Zero-Order Hold1/1
  Zero-Order Hold/1 -> Gain2/1
  Zero-Order Hold1/1 -> Gain3/1
  connections:
  PS-Simulink Converter/LConn1 -- s_trq_R/RConn1
  PS-Simulink Converter1/LConn1 -- s_trq_L/RConn1

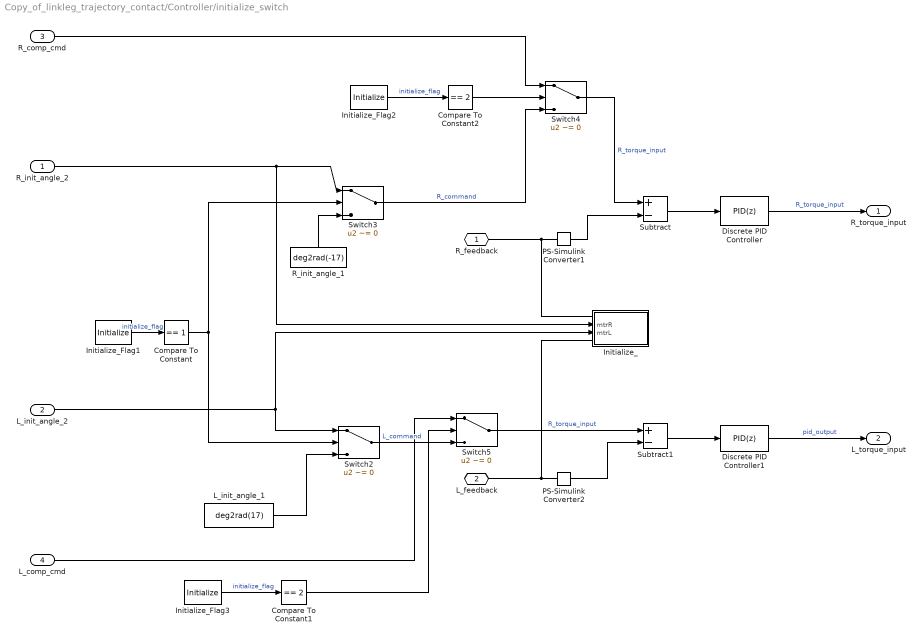
== system Copy_of_linkleg_trajectory_contact/Controller/initialize_switch ==
  R_init_angle_2 : Inport
  L_init_angle_2 : Inport  Port=2
  R_comp_cmd : Inport  Port=3
  L_comp_cmd : Inport  Port=4
  Compare To Constant : simulink/Logic and Bit Operations/Compare To Constant  relop===  const=1  OutDataTypeStr=boolean
  Compare To Constant1 : simulink/Logic and Bit Operations/Compare To Constant  relop===  const=2  OutDataTypeStr=uint8
  Compare To Constant2 : simulink/Logic and Bit Operations/Compare To Constant  relop===  const=2  OutDataTypeStr=uint8
  Discrete PID Controller : slpidlib/PID Controller  Controller=PID  Form=Parallel  TimeDomain=Discrete-time  UseExternalTs=off  SampleTime=-1  IntegratorMethod=Forward Euler  FilterMethod=Forward Euler  ControllerParametersSource=internal  P=50  I=0.02  UseKiTs=on  D=1.75  N=100  UseFilter=on  TunerSelectOption=Transfer Function Based (PID Tuner App)  InitialConditionSource=internal  InitialConditionForIntegrator=0  InitialConditionForFilter=0  DifferentiatorICPrevScaledInput=0  ExternalReset=none  TrackingMode=off  Kt=1  LimitOutput=on  SatLimitsSource=internal  UpperSaturationLimit=20  LowerSaturationLimit=-20  LinearizeAsGain=off  AntiWindupMode=none  Kb=1  LimitIntegrator=off  UpperIntegratorSaturationLimit=inf  LowerIntegratorSaturationLimit=-inf  POutMin=[]  POutMax=[]  IOutMin=[]  IOutMax=[]  DOutMin=[]  DOutMax=[]  NOutMin=[]  NOutMax=[]  SumOutMin=[]  SumOutMax=[]  SaturationOutMin=[]  SaturationOutMax=[]  PParamMin=[]  PParamMax=[]  IParamMin=[]  IParamMax=[]  DParamMin=[]  DParamMax=[]  NParamMin=[]  NParamMax=[]  KbParamMin=[]  KbParamMax=[]  KtParamMin=[]  KtParamMax=[]  KbOutMin=[]  KbOutMax=[]  KtOutMin=[]  KtOutMax=[]  IntegratorOutMin=[]  IntegratorOutMax=[]  FilterOutMin=[]  FilterOutMax=[]  SumI1OutMin=[]  SumI1OutMax=[]  SumI2OutMin=[]  SumI2OutMax=[]  SumI3OutMin=[]  SumI3OutMax=[]  SumI4OutMin=[]  SumI4OutMax=[]  SumDOutMin=[]  SumDOutMax=[]  DifferentiatorOutMin=[]  DifferentiatorOutMax=[]  FilterDiffOutCoefMin=[]  FilterDiffOutCoefMax=[]  ReciprocalOutMin=[]  ReciprocalOutMax=[]  SumDenOutMin=[]  SumDenOutMax=[]  SumNumOutMin=[]  SumNumOutMax=[]  DivideOutMin=[]  DivideOutMax=[]  UdiffTsProdOutMin=[]  UdiffTsProdOutMax=[]  NTsProdOutMin=[]  NTsProdOutMax=[]  UintegralTsProdOutMin=[]  UintegralTsProdOutMax=[]  UngainTsProdOutMin=[]  UngainTsProdOutMax=[]  ClampingZeroOutDataTypeStr=Inherit: Inherit via back propagation  ClampingZeroOutMin=[]  ClampingZeroOutMax=[]  FilterDenConstantOutDataTypeStr=Inherit: Inherit via back propagation  FilterDenConstantOutMin=[]  FilterDenConstantOutMax=[]  PCopyOutDataTypeStr=Inherit: Inherit via back propagation  PCopyOutMin=[]  PCopyOutMax=[]  NCopyOutDataTypeStr=Inherit: Inherit via back propagation  NCopyOutMin=[]  NCopyOutMax=[]  IntegratorContinuousStateAttributes=''  IntegratorStateMustResolveToSignalObject=off  IntegratorRTWStateStorageClass=Auto  FilterContinuousStateAttributes=''  FilterStateMustResolveToSignalObject=off  FilterRTWStateStorageClass=Auto  ParallelPVariant=InternalParameters  IdealPVariant=Disabled  IVariant=InternalParameters  DVariant=InternalParameters  IntegratorVariant=Discrete  SatVariant=Enabled  AWVariant=Passthrough  PCopyVariant=Disabled  TRVariant=Disabled  FdbkBlocksVariant=Forward  IdealPFdbkVariant=Disabled  SatFdbkVariant=Disabled  DerivativeFilterVariant=ForwardEulerFilter  NVariant=InternalParameters  NCopyVariant=Disabled  FilterICVariant=InternalICsFilter  IntegratorICVariant=InternalICs  ExternalResetVariant=Disabled  TRSumVariant=Passthrough  SumFdbkVariant=Disabled  SumVariant=Sum_PID  TsampFilterVariant=InternalTs  TsampNgainVariant=Passthrough  TsampIntegralVariant=Passthrough  ExternalSaturationOutDataTypeStr=Inherit: Same as second input
      settings: LibrarySourceBlock=simulink/Discrete/Discrete PID Controller
  Discrete PID Controller1 : slpidlib/PID Controller  Controller=PID  Form=Parallel  TimeDomain=Discrete-time  UseExternalTs=off  SampleTime=-1  IntegratorMethod=Forward Euler  FilterMethod=Forward Euler  ControllerParametersSource=internal  P=50  I=0.02  UseKiTs=on  D=1.75  N=100  UseFilter=on  TunerSelectOption=Transfer Function Based (PID Tuner App)  InitialConditionSource=internal  InitialConditionForIntegrator=0  InitialConditionForFilter=0  DifferentiatorICPrevScaledInput=0  ExternalReset=none  TrackingMode=off  Kt=1  LimitOutput=on  SatLimitsSource=internal  UpperSaturationLimit=20  LowerSaturationLimit=-20  LinearizeAsGain=off  AntiWindupMode=none  Kb=1  LimitIntegrator=off  UpperIntegratorSaturationLimit=inf  LowerIntegratorSaturationLimit=-inf  POutMin=[]  POutMax=[]  IOutMin=[]  IOutMax=[]  DOutMin=[]  DOutMax=[]  NOutMin=[]  NOutMax=[]  SumOutMin=[]  SumOutMax=[]  SaturationOutMin=[]  SaturationOutMax=[]  PParamMin=[]  PParamMax=[]  IParamMin=[]  IParamMax=[]  DParamMin=[]  DParamMax=[]  NParamMin=[]  NParamMax=[]  KbParamMin=[]  KbParamMax=[]  KtParamMin=[]  KtParamMax=[]  KbOutMin=[]  KbOutMax=[]  KtOutMin=[]  KtOutMax=[]  IntegratorOutMin=[]  IntegratorOutMax=[]  FilterOutMin=[]  FilterOutMax=[]  SumI1OutMin=[]  SumI1OutMax=[]  SumI2OutMin=[]  SumI2OutMax=[]  SumI3OutMin=[]  SumI3OutMax=[]  SumI4OutMin=[]  SumI4OutMax=[]  SumDOutMin=[]  SumDOutMax=[]  DifferentiatorOutMin=[]  DifferentiatorOutMax=[]  FilterDiffOutCoefMin=[]  FilterDiffOutCoefMax=[]  ReciprocalOutMin=[]  ReciprocalOutMax=[]  SumDenOutMin=[]  SumDenOutMax=[]  SumNumOutMin=[]  SumNumOutMax=[]  DivideOutMin=[]  DivideOutMax=[]  UdiffTsProdOutMin=[]  UdiffTsProdOutMax=[]  NTsProdOutMin=[]  NTsProdOutMax=[]  UintegralTsProdOutMin=[]  UintegralTsProdOutMax=[]  UngainTsProdOutMin=[]  UngainTsProdOutMax=[]  ClampingZeroOutDataTypeStr=Inherit: Inherit via back propagation  ClampingZeroOutMin=[]  ClampingZeroOutMax=[]  FilterDenConstantOutDataTypeStr=Inherit: Inherit via back propagation  FilterDenConstantOutMin=[]  FilterDenConstantOutMax=[]  PCopyOutDataTypeStr=Inherit: Inherit via back propagation  PCopyOutMin=[]  PCopyOutMax=[]  NCopyOutDataTypeStr=Inherit: Inherit via back propagation  NCopyOutMin=[]  NCopyOutMax=[]  IntegratorContinuousStateAttributes=''  IntegratorStateMustResolveToSignalObject=off  IntegratorRTWStateStorageClass=Auto  FilterContinuousStateAttributes=''  FilterStateMustResolveToSignalObject=off  FilterRTWStateStorageClass=Auto  ParallelPVariant=InternalParameters  IdealPVariant=Disabled  IVariant=InternalParameters  DVariant=InternalParameters  IntegratorVariant=Discrete  SatVariant=Enabled  AWVariant=Passthrough  PCopyVariant=Disabled  TRVariant=Disabled  FdbkBlocksVariant=Forward  IdealPFdbkVariant=Disabled  SatFdbkVariant=Disabled  DerivativeFilterVariant=ForwardEulerFilter  NVariant=InternalParameters  NCopyVariant=Disabled  FilterICVariant=InternalICsFilter  IntegratorICVariant=InternalICs  ExternalResetVariant=Disabled  TRSumVariant=Passthrough  SumFdbkVariant=Disabled  SumVariant=Sum_PID  TsampFilterVariant=InternalTs  TsampNgainVariant=Passthrough  TsampIntegralVariant=Passthrough  ExternalSaturationOutDataTypeStr=Inherit: Same as second input
      settings: LibrarySourceBlock=simulink/Discrete/Discrete PID Controller
  Initialize_ : Subsystem
      settings: PortSchema="{\"entries\":[{\"content\":{\"sides\":[{\"content\":{\"connectorIds\":[\"LConn1\",\"In1\",\"In2\",\"LConn2\"]},\"type\":\"ConnectorPlacement.EquallySpacedRectSide\",\"uuid\":\"a1447eaf-58b1-44c6-851b-614a5a67ef95\"},{\"content\":{\"connectorIds\":[],\"side\":\"RIGHT\"},\"type\":\"ConnectorPlacement.EquallySpacedRectSide\",\"uuid\":\"571935e7-f70b-4c6f-917a-79f73ad389fd\"},{\"content\":{\"connectorIds\":[],\"side\":\"TOP\"},\"type\":\"ConnectorPlacement.EquallySpacedRectSide\",\"uuid\":\"5a070d43-0df0-4350-9269-167e1f7fd924\"}]},\"type\":\"ConnectorPlacement.EquallySpacedConnector\",\"uuid\":\"e4886c4e-8163-4194-b7e2-d337b7ad029a\"}],\"packageUris\":[\"http://schema.mathworks.com/mf0/Connector/R2020b\"],\"version\":\"1.0\"}"
  Initialize_Flag1 : DataStoreRead  DataStoreName=Initialize  IndexOptions=Index vector (dialog)  Indices=1  OutputSizes=1
  Initialize_Flag2 : DataStoreRead  DataStoreName=Initialize  IndexOptions=Index vector (dialog)  Indices=1  OutputSizes=1
  Initialize_Flag3 : DataStoreRead  DataStoreName=Initialize  IndexOptions=Index vector (dialog)  Indices=1  OutputSizes=1
  L_init_angle_1 : Constant  Value=deg2rad(17)
  PS-Simulink Converter1 : nesl_utility/PS-Simulink Converter  PhysicalDomain=network_engine_domain  SubClassName=ps_output  LeftPortType=input  RightPortType=output  PseudoPeriodic=off  Frequencies=[]  VectorFormat=inherit  Unit=inherit  AffineConversion=off
  PS-Simulink Converter2 : nesl_utility/PS-Simulink Converter  PhysicalDomain=network_engine_domain  SubClassName=ps_output  LeftPortType=input  RightPortType=output  PseudoPeriodic=off  Frequencies=[]  VectorFormat=inherit  Unit=inherit  AffineConversion=off
  R_init_angle_1 : Constant  Value=deg2rad(-17)
  Subtract : Sum  Inputs=+-
  Subtract1 : Sum  Inputs=+-
  Switch{2..5} (4 alike) : Switch  Criteria=u2 ~= 0  Threshold=0.5  SaturateOnIntegerOverflow=off  InputSameDT=off
  R_feedback : PMIOPort  Side=Left
  L_feedback : PMIOPort  Port=2  Side=Left
  R_torque_input : Outport
  L_torque_input : Outport  Port=2
  wires:
  Discrete PID Controller/1 -> R_torque_input/1  "R_torque_input"
  Subtract/1 -> Discrete PID Controller/1
  PS-Simulink Converter2/1 -> Subtract1/2
  Initialize_Flag1/1 -> Compare To Constant/1  "initialize_flag"
  R_init_angle_1/1 -> Switch3/3
  PS-Simulink Converter1/1 -> Subtract/2
  L_init_angle_2/1 -> Initialize_/2(mtrL), Switch2/1
  R_init_angle_2/1 -> Switch3/1, Initialize_/1(mtrR)
  L_init_angle_1/1 -> Switch2/3
  Compare To Constant/1 -> Switch3/2, Switch2/2
  Switch2/1 -> Switch5/3  "L_command"
  Subtract1/1 -> Discrete PID Controller1/1
  Initialize_Flag2/1 -> Compare To Constant2/1  "initialize_flag"
  Compare To Constant2/1 -> Switch4/2
  Switch3/1 -> Switch4/3  "R_command"
  Switch4/1 -> Subtract/1  "R_torque_input"
  R_comp_cmd/1 -> Switch4/1
  Initialize_Flag3/1 -> Compare To Constant1/1  "initialize_flag"
  Compare To Constant1/1 -> Switch5/2
  Switch5/1 -> Subtract1/1  "R_torque_input"
  Discrete PID Controller1/1 -> L_torque_input/1  "pid_output"
  L_comp_cmd/1 -> Switch5/1
  connections:
  PS-Simulink Converter1/LConn1 -- R_feedback/RConn1 -- Initialize_/LConn1
  PS-Simulink Converter2/LConn1 -- L_feedback/RConn1 -- Initialize_/LConn2

== system Copy_of_linkleg_trajectory_contact/Controller/tb_delay ==
  tb : Inport
  Delay : Delay
  Delay1 : Delay  DelayLength=1
  Delay2 : Delay  DelayLength=3
  Mux : Mux
  Out1 : Outport
  wires:
  Delay1/1 -> Mux/2
  Delay/1 -> Mux/3
  tb/1 -> Delay2/1, Delay/1, Delay1/1, Mux/1
  Mux/1 -> Out1/1
  Delay2/1 -> Mux/4

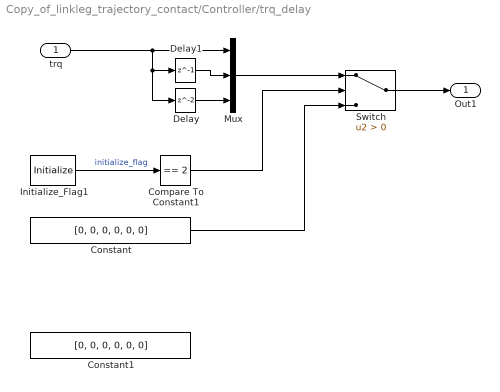
== system Copy_of_linkleg_trajectory_contact/Controller/trq_delay ==
  trq : Inport
  Compare To Constant1 : simulink/Logic and Bit Operations/Compare To Constant  relop===  const=2  OutDataTypeStr=uint8
  Constant : Constant  Value=[0, 0, 0, 0, 0, 0]
  Constant1 : Constant  Value=[0, 0, 0, 0, 0, 0]
  Delay : Delay
  Delay1 : Delay  DelayLength=1
  Initialize_Flag1 : DataStoreRead  DataStoreName=Initialize  IndexOptions=Index vector (dialog)  Indices=1  OutputSizes=1
  Mux : Mux  Inputs=3
  Switch : Switch  Criteria=u2 > Threshold  SaturateOnIntegerOverflow=off  InputSameDT=off
  Out1 : Outport
  wires:
  trq/1 -> Delay1/1, Delay/1, Mux/1
  Delay/1 -> Mux/3
  Delay1/1 -> Mux/2
  Compare To Constant1/1 -> Switch/2
  Initialize_Flag1/1 -> Compare To Constant1/1  "initialize_flag"
  Switch/1 -> Out1/1
  Mux/1 -> Switch/1
  Constant/1 -> Switch/3

== system Copy_of_linkleg_trajectory_contact/Controller/x_ref_delay ==
  In1 : Inport
  In2 : Inport  Port=2
  Delay : Delay
  Delay1 : Delay
  Delay2 : Delay  DelayLength=1
  Delay3 : Delay  DelayLength=1
  Mux2 : Mux  Inputs=6
  x_des : Outport
  wires:
  Delay1/1 -> Mux2/6
  Mux2/1 -> x_des/1  "x_des"
  Delay3/1 -> Mux2/3
  Delay/1 -> Mux2/5
  Delay2/1 -> Mux2/4
  In2/1 -> Delay1/1, Delay2/1, Mux2/2
  In1/1 -> Delay/1, Delay3/1, Mux2/1

== system Copy_of_linkleg_trajectory_contact/Controller/xc_delay ==
  In1 : Inport
  Compare To Constant1 : simulink/Logic and Bit Operations/Compare To Constant  relop===  const=2  OutDataTypeStr=uint8
  Constant : Constant  Value=[-0.1, -0.15, -0.1, -0.15]
  Constant1 : Constant  Value=[-0.1, -0.22, -0.1, -0.22]
  Delay : Delay  DelayLength=1
  Delay1 : Delay
  Initialize_Flag1 : DataStoreRead  DataStoreName=Initialize  IndexOptions=Index vector (dialog)  Indices=1  OutputSizes=1
  Mux1 : Mux  Inputs=2
  Switch : Switch  Criteria=u2 > Threshold  SaturateOnIntegerOverflow=off  InputSameDT=off
  X_c : Outport
  wires:
  Delay/1 -> Mux1/1
  Delay1/1 -> Mux1/2
  In1/1 -> Delay/1, Delay1/1
  Initialize_Flag1/1 -> Compare To Constant1/1  "initialize_flag"
  Switch/1 -> X_c/1
  Compare To Constant1/1 -> Switch/2
  Mux1/1 -> Switch/1  "X_c"
  Constant/1 -> Switch/3
